simulink model "simulacion_tres_tanques"  (R2012b)
settings: Solver=ode45  StartTime=0.0  StopTime=10.0  RelTol=1e-3
settings Model: CovModelRefEnable=off  Creator=nico  LastModifiedBy=nico
settings DataIOCC: SaveFormat=StructureWithTime
settings OptimizationCC: ExpressionDepthLimit=128
settings DebuggingCC: UnderspecifiedInitializationDetection=Simplified  MergeDetectMultiDrivingBlocksExec=error  SolverPrmCheckMsg=none  FrameProcessingCompatibilityMsg=error  StateNameClashWarn=none
settings HardwareCC: ProdBitPerPointer=64  ProdLargestAtomicFloat=Float  ProdIntDivRoundTo=Zero  ProdEndianess=LittleEndian  ProdHWDeviceType=Specified
settings CodeAppCC: CustomSymbolStrType=$N$R$M_T
settings GRTTargetCC: CodeReplacementLibrary=C89/C90 (ANSI)  GeneratePreprocessorConditionals=Use local settings

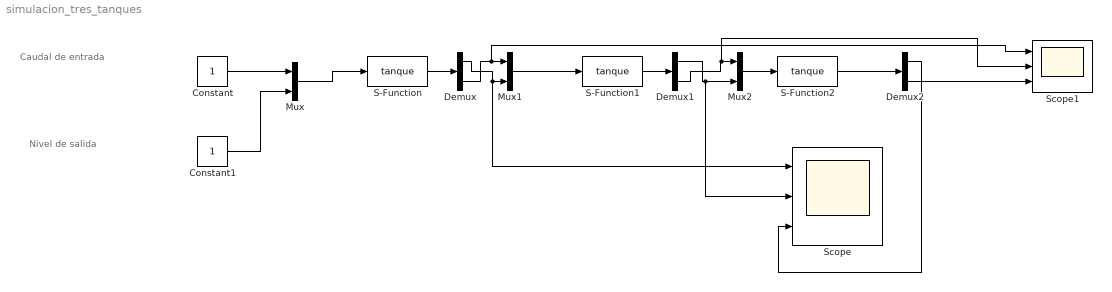
== system simulacion_tres_tanques ==
  note: Nivel de salida
  note: Caudal de entrada
  Constant : Constant
  Constant1 : Constant
  Demux : Demux  Outputs=2
  Demux1 : Demux  Outputs=2
  Demux2 : Demux  Outputs=2
  Mux : Mux  Inputs=2
  Mux1 : Mux  Inputs=2
  Mux2 : Mux  Inputs=2
  S-Function : S-Function  FunctionName=tanque  Parameters=1 8 1 5  SFunctionDeploymentMode=off  EnableBusSupport=off
  S-Function1 : S-Function  FunctionName=tanque  Parameters=1 8 1 3  SFunctionDeploymentMode=off  EnableBusSupport=off
  S-Function2 : S-Function  FunctionName=tanque  Parameters=10 8 1 6  SFunctionDeploymentMode=off  EnableBusSupport=off
  Scope : Scope  NumInputPorts=3
      settings: TimeRange=auto  MaxDataPoints=5000  SaveToWorkspace=off  SaveName=ScopeData  YMin=1.29084~-5~-5  YMax=8.74546~5~5  SampleTime=-1
  Scope1 : Scope  NumInputPorts=3
      settings: TimeRange=auto  MaxDataPoints=5000  SaveToWorkspace=off  YMin=0.00156~-5~-5  YMax=2.22205~5~5  SampleTime=-1
  wires:
  Constant/1 -> Mux/1
  Mux/1 -> S-Function/1
  Constant1/1 -> Mux/2
  S-Function/1 -> Demux/1
  Demux/2 -> Scope1/1, Mux1/1
  Demux/1 -> Scope/1, Mux1/2
  Mux1/1 -> S-Function1/1
  Mux2/1 -> S-Function2/1
  S-Function1/1 -> Demux1/1
  Demux1/1 -> Scope/2, Mux2/2
  Demux1/2 -> Scope1/2, Mux2/1
  S-Function2/1 -> Demux2/1
  Demux2/1 -> Scope/3
  Demux2/2 -> Scope1/3
